simulink model "sim_topic2"  (R2023b)
settings: Solver=FixedStepAuto  StartTime=0.0  StopTime=T_sim  FixedStep=dt_sim  RelTol=1e-3
undefined symbols (not defined in the file): den_Cd_tf, den_Gp_tf, num_Cd_tf, num_Gp_tf, omega_d, T
settings Model: Creator=user  LastModifiedBy=user

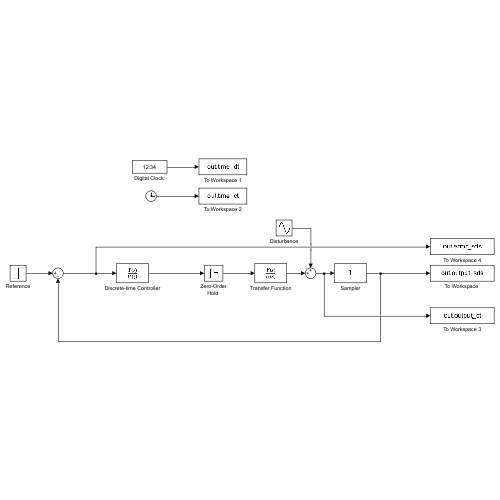
[thumbnail: Simulink's stored preview of the top-level diagram]
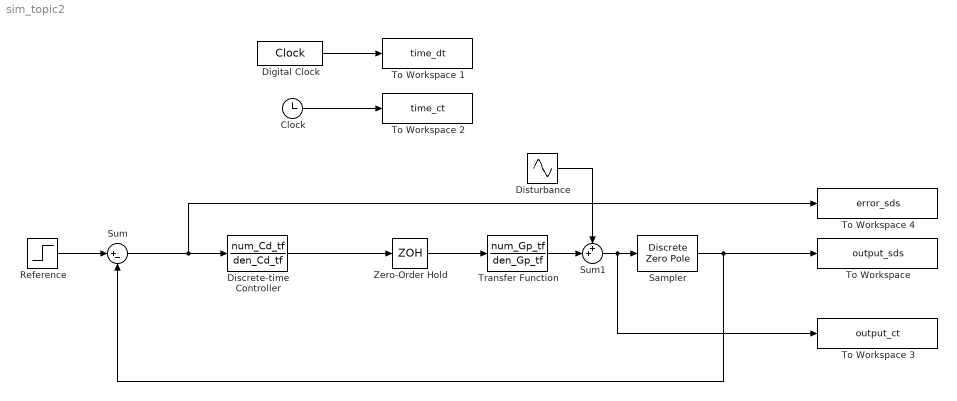
== system sim_topic2 ==
  Clock : Clock
  "Digital Clock " : DigitalClock  SampleTime=T
  Discrete-time Controller : DiscreteTransferFcn  Numerator=num_Cd_tf  Denominator=den_Cd_tf
  Disturbance : Sin  Amplitude=0.2  Frequency=omega_d  SampleTime=0
  Reference : Step  Time=0  SampleTime=T
  Sampler : DiscreteZeroPole  Zeros=[]  Poles=[]  Gain=1  SampleTime=T
  Sum : Sum  Inputs=|+-
  Sum1 : Sum  Inputs=++|
  "To Workspace " : ToWorkspace  VariableName=output_sds  SampleTime=T
  To Workspace 1 : ToWorkspace  VariableName=time_dt  SampleTime=T
  To Workspace 2 : ToWorkspace  VariableName=time_ct  SampleTime=-1
  To Workspace 3 : ToWorkspace  VariableName=output_ct  SampleTime=-1
  To Workspace 4 : ToWorkspace  VariableName=error_sds  SampleTime=T
  Transfer Function : TransferFcn  Numerator=num_Gp_tf  Denominator=den_Gp_tf
  "Zero-Order Hold " : ZeroOrderHold  SampleTime=-1
  wires:
  Clock/1 -> To Workspace 2/1
  "Zero-Order Hold "/1 -> Transfer Function/1
  "Digital Clock "/1 -> To Workspace 1/1
  Sampler/1 -> "To Workspace "/1, Sum/2
  Reference/1 -> Sum/1
  Sum/1 -> To Workspace 4/1, Discrete-time Controller/1
  Discrete-time Controller/1 -> "Zero-Order Hold "/1
  Sum1/1 -> To Workspace 3/1, Sampler/1
  Transfer Function/1 -> Sum1/2
  Disturbance/1 -> Sum1/1
